simulink model "Dsss"  (R2023b)
settings: Solver=VariableStepAuto  StartTime=0.0  StopTime=2e-3  RelTol=1e-3
libraries: simulink x1
settings Model: Creator=Dell  LastModifiedBy=Dell

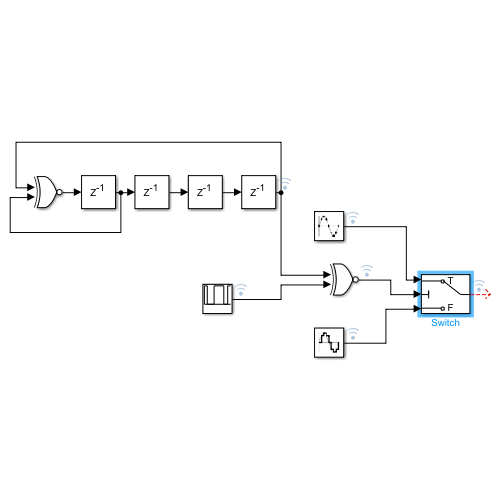
[thumbnail: Simulink's stored preview of the top-level diagram]
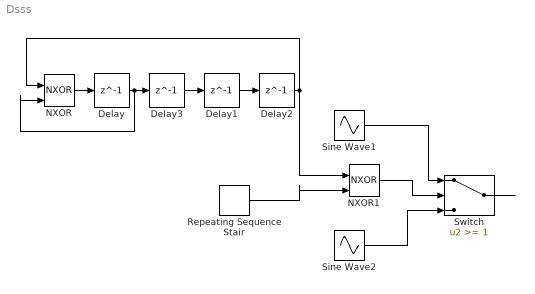
== system Dsss ==
  Delay{,1..3} (4 alike) : Delay  DelayLength=1  InitialCondition=0  SampleTime=10e-6
  NXOR : Logic  Operator=NXOR  IconShape=distinctive  AllPortsSameDT=off  OutDataTypeStr=boolean
  NXOR1 : Logic  Operator=NXOR  IconShape=distinctive  AllPortsSameDT=off  OutDataTypeStr=boolean
  Repeating Sequence Stair : simulink/Sources/Repeating Sequence Stair  OutValues=[1 0 0 1 1 1 0 1].'  tsamp=150e-6  OutMin=[]  OutMax=[]  OutDataTypeStr=double  OutputDataTypeScalingMode=double  OutDataType=fixdt(0,8)  ConRadixGroup=Best Precision: Vector-wise  OutScaling=2^-12
  Sine Wave1 : Sin  SineType=Sample based  Frequency=700000  Samples=36  SampleTime=40e-9
  Sine Wave2 : Sin  Frequency=2*pi*694e3  Phase=pi  Samples=36  SampleTime=40e-9
  Switch : Switch  Threshold=1  SaturateOnIntegerOverflow=off  InputSameDT=off
  wires:
  Delay3/1 -> Delay1/1
  Delay1/1 -> Delay2/1
  Delay/1 -> NXOR/2, Delay3/1
  NXOR/1 -> Delay/1
  Delay2/1 -> NXOR/1, NXOR1/1
  Repeating Sequence Stair/1 -> NXOR1/2
  NXOR1/1 -> Switch/2
  Sine Wave1/1 -> Switch/1
  Sine Wave2/1 -> Switch/3
  Switch/1 -> ?
